simulink library "NXTFcns"  (R2014b)
settings: Solver=ode45  StartTime=0.0  StopTime=10.0  RelTol=1e-3
libraries: legonxtlib x2
settings Model: Creator=pvinnako  LastModifiedBy=pvinnako

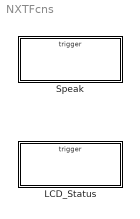
== system NXTFcns ==
  LCD_Status : Subsystem  TreatAsAtomicUnit=on
  Speak : Subsystem  TreatAsAtomicUnit=on

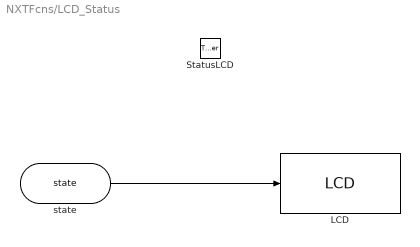
== system NXTFcns/LCD_Status ==
  StatusLCD : TriggerPort  TriggerType=function-call  IsSimulinkFunction=on  FunctionName=StatusLCD
  LCD : legonxtlib/LCD  slcdStr=Status  slcdLine=1  slcdFormat=Decimal
  state : ArgIn  ArgumentName=state
  wires:
  state/1 -> LCD/1

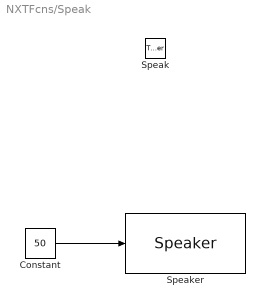
== system NXTFcns/Speak ==
  Speak : TriggerPort  TriggerType=function-call  IsSimulinkFunction=on  FunctionName=Speak
  Constant : Constant  Value=50
  Speaker : legonxtlib/Speaker  sinputMode=Volume only  sspeakerFreq=800  sspeakerVolume=50  sspeakerDuration=100
  wires:
  Constant/1 -> Speaker/1
